simulink model "pcssp_gas_pipe"  (R2020b)
settings: Solver=VariableStepAuto  StartTime=0.0  StopTime=10.0  RelTol=1e-3
model mask{pcssp_gas_pipe_fp_shape=pcssp_gas_pipe_fp_shape}
model workspace (MAT data in the model file):
  pcssp_gas_pipe_fp_shape.port = 3
  pcssp_gas_pipe_fp_shape.position = 1
  pcssp_gas_pipe_fp_shape.length = 30.8
  pcssp_gas_pipe_fp_shape.R0 = 0.00635
  pcssp_gas_pipe_fp_shape.N = 20
  pcssp_gas_pipe_fp_shape.Katan = 100000
  pcssp_gas_pipe_fp_shape.Cp = 1
  pcssp_gas_pipe_fp_shape.Temp = 343.15
  pcssp_gas_pipe_fp_shape.bnd_cond_mode = 1
  pcssp_gas_pipe_fp_shape.AM = [0 0 0 0 0 0 0 0 0 0 0 0 ... (1600 elements, 40x40)]
  pcssp_gas_pipe_fp_shape.BM = [-1  0; 0  0; 0  0; 0  0; 0  0; 0  0; 0  0; 0  0; 0  0; 0  0; 0  0; 0  0; 0  0; 0  0; 0  0; 0  0; 0  0; 0  0; 0  0; 0  0; 0  0; 0  0; 0  0; 0  0; 0  0; 0  0; 0  0; 0  0; 0  0; 0  0; 0  0; 0  0; 0  0; 0  0; 0  0; 0  0; 0  0; 0  0; 0  0; 0  1]
  pcssp_gas_pipe_fp_shape.CM = [1  0  0  0  0  0  0  0  0  0  0  0  0  0  0  0  0  0  0  0  0  0  0  0  0  0  0  0  0  0  0  0  0  0  0  0  0  0  0  0; 0  0  0  0  0  0  0  0  0  0  0  0  0  0  0  0  0  0  0  0  0  0  0  0  0  0  0  0  0  0  0  0  0  0  0  0  0  0  0  1]
  pcssp_gas_pipe_fp_shape.dx = 1.62105263158
  pcssp_gas_pipe_fp_shape.d = 0.0127
  pcssp_gas_pipe_fp_shape.A = 0.000126676869774
  pcssp_gas_pipe_fp_shape.gamma = 1.4
  pcssp_gas_pipe_fp_shape.C1 = [7.28871016193e-05  7.28871016193e-05  0  0  0  0  0  0  0  0  0  0  0  0  0  0  0  0  0  0; 0  7.28871016193e-05  7.28871016193e-05  0  0  0  0  0  0  0  0  0  0  0  0  0  0  0  0  0; 0  0  7.28871016193e-05  7.28871016193e-05  0  0  0  0  0  0  0  0  0  0  0  0  0  0  0  0; 0  0  0  7.28871016193e-05  7.28871016193e-05  0  0  0  0  0  0  0  0  0  0  0  0  0  0  0; 0  0  0  0  7.28871016193e-05  7.28871016193e-05  0  0  0  0  0  0  0  0  0  0  0  0  0  0; 0  0  0  0  0  7.28871016193e-05  7.28871016193e-05  0  0  0  0  0  0  0  0  0  0  0  0  0; 0  0  0  0  0  0  7.28871016193e-05  7.28871016193e-05  0  0  0  0  0  0  0  0  0  0  0  0; 0  0  0  0  0  0  0  7.28871016193e-05  7.28871016193e-05  0  0  0  0  0  0  0  0  0  0  0; 0  0  0  0  0  0  0  0  7.28871016193e-05  7.28871016193e-05  0  0  0  0  0  0  0  0  0  0; 0  0  0  0  0  0  0  0  0  7.28871016193e-05  7.28871016193e-05  0  0  0  0  0  0  0  0  0; 0  0  0  0  0  0  0  0  0  0  7.28871016193e-05  7.28871016193e-05  0  0  0  0  0  0  0  0; 0  0  0  0  0  0  0  0  0  0  0  7.28871016193e-05  7.28871016193e-05  0  0  0  0  0  0  0; 0  0  0  0  0  0  0  0  0  0  0  0  7.28871016193e-05  7.28871016193e-05  0  0  0  0  0  0; 0  0  0  0  0  0  0  0  0  0  0  0  0  7.28871016193e-05  7.28871016193e-05  0  0  0  0  0; 0  0  0  0  0  0  0  0  0  0  0  0  0  0  7.28871016193e-05  7.28871016193e-05  0  0  0  0; 0  0  0  0  0  0  0  0  0  0  0  0  0  0  0  7.28871016193e-05  7.28871016193e-05  0  0  0; 0  0  0  0  0  0  0  0  0  0  0  0  0  0  0  0  7.28871016193e-05  7.28871016193e-05  0  0; 0  0  0  0  0  0  0  0  0  0  0  0  0  0  0  0  0  7.28871016193e-05  7.28871016193e-05  0; 0  0  0  0  0  0  0  0  0  0  0  0  0  0  0  0  0  0  7.28871016193e-05  7.28871016193e-05; 0  0  0  0  0  0  0  0  0  0  0  0  0  0  0  0  0  0  0  0]
  pcssp_gas_pipe_fp_shape.C1out = 2.24814112137e-05
undefined symbols (not defined in the file or in its folder): AM, BM, config, dx, pcssp_gas_pipe, pcssp_gas_pipe_fp
libraries: PCSSP_iter_actuator_modules x2
settings Model: DataDictionary=pcssp_gas_pipe.sldd  ParameterArgumentNames=pcssp_gas_pipe_fp_shape  OrderedModelArguments=off  Creator=ravenst1  LastModifiedBy=ravenst1

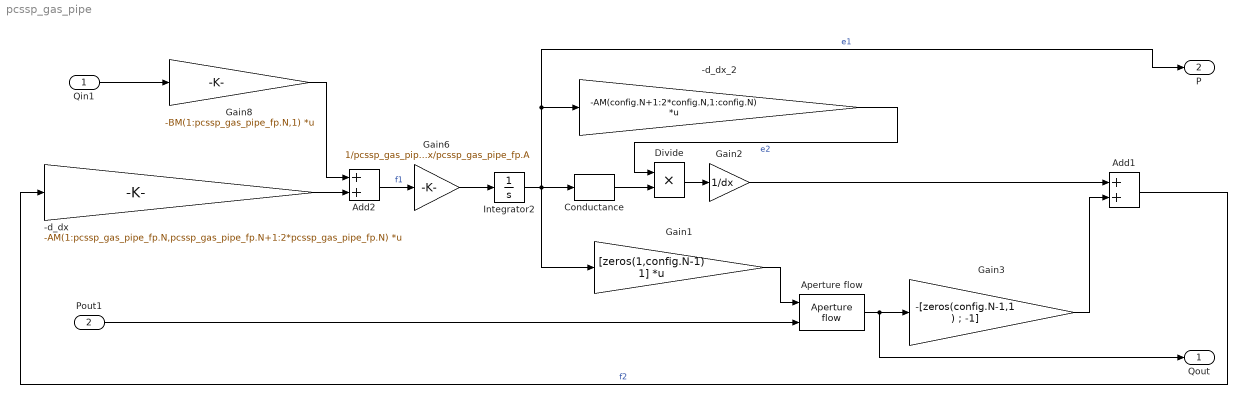
== system pcssp_gas_pipe ==
  Qin1 : Inport
  Pout1 : Inport  Port=2
  -d_dx : Gain  Gain=-AM(1:pcssp_gas_pipe_fp.N,pcssp_gas_pipe_fp.N+1:2*pcssp_gas_pipe_fp.N)  Multiplication=Matrix(K*u)
  -d_dx_2 : Gain  Gain=-AM(config.N+1:2*config.N,1:config.N)  Multiplication=Matrix(K*u)
  Add1 : Sum
  Add2 : Sum
  Aperture flow : PCSSP_iter_actuator_modules/GasPipe/Aperture flow  SystemSampleTime=-1  VariantActivationTime=update diagram  Latency=0  AutoFrameSizeCalculation=off
  Conductance : PCSSP_iter_actuator_modules/GasPipe/Conductance  SystemSampleTime=-1  VariantActivationTime=update diagram  Latency=0  AutoFrameSizeCalculation=off
  Divide : Product  Inputs=**
  Gain1 : Gain  Gain=[zeros(1,config.N-1) 1]  Multiplication=Matrix(K*u)
  Gain2 : Gain  Gain=1/dx
  Gain3 : Gain  Gain=-[zeros(config.N-1,1 ) ; -1]
  Gain6 : Gain  Gain=1/pcssp_gas_pipe_fp.dx/pcssp_gas_pipe_fp.A
  Gain8 : Gain  Gain=-BM(1:pcssp_gas_pipe_fp.N,1)  Multiplication=Matrix(K*u)
  Integrator2 : Integrator  InitialCondition=pcssp_gas_pipe.p0
  Qout : Outport
  P : Outport  Port=2
  wires:
  Add1/1 -> -d_dx/1  "f2"
  Aperture flow/1 -> Qout/1, Gain3/1
  Gain3/1 -> Add1/2
  Conductance/1 -> Divide/2
  Gain1/1 -> Aperture flow/1
  Add2/1 -> Gain6/1  "f1"
  Divide/1 -> Gain2/1
  Gain2/1 -> Add1/1
  Qin1/1 -> Gain8/1
  Integrator2/1 -> P/1, -d_dx_2/1, Gain1/1, Conductance/1  "e1"
  Pout1/1 -> Aperture flow/2
  Gain8/1 -> Add2/1
  -d_dx/1 -> Add2/2
  Gain6/1 -> Integrator2/1
  -d_dx_2/1 -> Divide/1  "e2"
